simulink model "verifica_tensione"  (R2014a)
settings: Solver=ode45  StartTime=0.0  StopTime=20.0  RelTol=1e-3
libraries: cstblocks x2, simulink x1
settings Model: Creator=UTENTE  LastModifiedBy=UTENTE

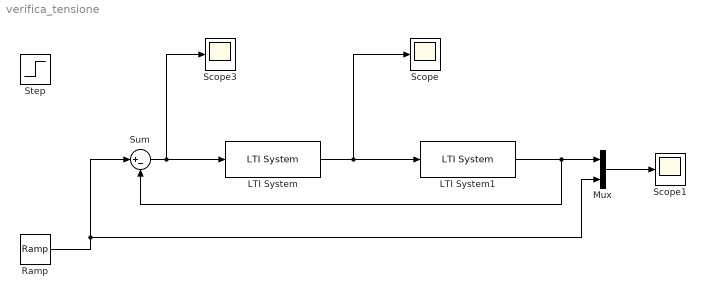
== system verifica_tensione ==
  LTI System : cstblocks/LTI System  sys=Cz1  IC=[]
  LTI System1 : cstblocks/LTI System  sys=Fz  IC=[]
  Mux : Mux  Inputs=2
  Ramp : simulink/Sources/Ramp  slope=1  start=0  X0=0
  Scope : Scope
  Scope1 : Scope
  Scope3 : Scope
      settings: SaveName=ScopeData3
  Step : Step  Time=0  SampleTime=0
  Sum : Sum  Inputs=|+-
  wires:
  Mux/1 -> Scope1/1
  Sum/1 -> Scope3/1, LTI System/1
  LTI System/1 -> Scope/1, LTI System1/1
  LTI System1/1 -> Sum/2, Mux/1
  Ramp/1 -> Mux/2, Sum/1
